simulink model "AtmLast2Real"  (R2015a)
settings: configuration reference "SIMULATION_CONFIGURATION" (kept outside this file)
settings Model: CovSFcnEnable=off  Creator=moritz  LastModifiedBy=moritz
settings ConfigSetRef: SourceLocation=Base Workspace

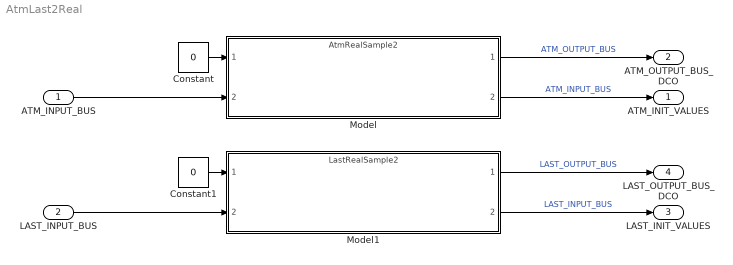
== system AtmLast2Real ==
  ATM_INPUT_BUS : Inport  OutDataTypeStr=Bus: ATM_INPUT_BUS  BusOutputAsStruct=on
  LAST_INPUT_BUS : Inport  Port=2  OutDataTypeStr=Bus: LAST_INPUT_BUS  BusOutputAsStruct=on
  Constant : Constant  Value=0  OutDataTypeStr=boolean
  Constant1 : Constant  Value=0  OutDataTypeStr=boolean
  Model : ModelReference  ModelNameDialog=AtmRealSample2  Variant=on  ModelReferenceVersion=1.17  DefaultDataLogging=on
  Model1 : ModelReference  ModelNameDialog=LastRealSample2  Variant=on  ModelReferenceVersion=1.20  DefaultDataLogging=on
  ATM_INIT_VALUES : Outport  OutDataTypeStr=Bus: ATM_INPUT_BUS  BusOutputAsStruct=on
  ATM_OUTPUT_BUS_DCO : Outport  Port=2  OutDataTypeStr=Bus: ATM_OUTPUT_BUS  BusOutputAsStruct=on
  LAST_INIT_VALUES : Outport  Port=3  OutDataTypeStr=Bus: LAST_INPUT_BUS  BusOutputAsStruct=on
  LAST_OUTPUT_BUS_DCO : Outport  Port=4  OutDataTypeStr=Bus: LAST_OUTPUT_BUS  BusOutputAsStruct=on
  wires:
  Model/1 -> ATM_OUTPUT_BUS_DCO/1  "ATM_OUTPUT_BUS"
  Model1/1 -> LAST_OUTPUT_BUS_DCO/1  "LAST_OUTPUT_BUS"
  Model/2 -> ATM_INIT_VALUES/1  "ATM_INPUT_BUS"
  Model1/2 -> LAST_INIT_VALUES/1  "LAST_INPUT_BUS"
  ATM_INPUT_BUS/1 -> Model/2
  LAST_INPUT_BUS/1 -> Model1/2
  Constant/1 -> Model/1
  Constant1/1 -> Model1/1
